simulink model "HC_core_control"  (R2023b)
settings: Solver=FixedStepAuto  StartTime=0.0  StopTime=inf  FixedStep=0.0002  RelTol=1e-4  AbsTol=1e-6
undefined symbols (not defined in the file): shuntMaxRequestedCurrentrms
settings Model: DataDictionary=fmuGenerationDictionay.sldd  ModifiedByFormat=Third Equation Ltd  Creator=Third Equation Ltd  LastModifiedBy=Third Equation Ltd
settings ConfigSet: Description=|
  | Fast task configuration for protected model and FMU generation
  | Sample frequency = 5000 Hz
settings SolverCC: AutoScaleAbsTol=off  AlgebraicLoopSolver=TrustRegion  MaxZcPerStep=1
settings DataIOCC: ExternalInput=[]  InitialState=[]  SaveFormat=Array  SaveOutput=off  SaveTime=off  ReturnWorkspaceOutputs=off
settings OptimizationCC: BlockReduction=off  BooleanDataType=off  ReuseModelBlockBuffer=off  ExpressionDepthLimit=2147483647  InitFltsAndDblsToZero=on
settings DebuggingCC: SaveWithParameterizedLinksMsg=none  SignalResolutionControl=TryResolveAllWithWarning  MultiTaskDSMMsg=warning  MultiTaskCondExecSysMsg=none  IntegerOverflowMsg=none  FcnCallInpInsideContextMsg=warning  UnconnectedInputMsg=warning  UnconnectedOutputMsg=warning  UnconnectedLineMsg=warning  StateNameClashWarn=warning  SFUnexpectedBacktrackingDiag=warning  SFNoUnconditionalDefaultTransitionDiag=warning  SFExecutionAtInitializationDiag=none  IntegerSaturationMsg=none  UnderSpecifiedDimensionMsg=warning  ArithmeticOperatorsInVariantConditions=warning
settings HardwareCC: ProdBitPerPointer=32  ProdBitPerSizeT=32  ProdBitPerPtrDiffT=32  ProdLargestAtomicFloat=None  ProdWordSize=32  ProdHWDeviceType=Custom Processor->Custom Processor
settings ModelReferenceCC: EnableRefExpFcnMdlSchedulingChecks=on  PropagateSignalLabelsOutOfModel=off
settings SFSimCC: SimUseLocalCustomCode=off  CustomCodeUndefinedFunction=UseInterfaceOnly
settings RTWCC: Description=FMU2CS  SystemTargetFile=fmu2cs.tlc  TemplateMakefile=fmu2cs_default_tmf  RTWUseLocalCustomCode=off  DLArmComputeVersion=19.05
settings CodeAppCC: StateflowObjectComments=on
settings GRTTargetCC: TargetLangStandard=C89/C90 (ANSI)  CombineOutputUpdateFcns=off  MatFileLogging=off
settings ConfigComp: CovMetricSettings=dw  CovSaveCumulativeToWorkspaceVar=on  CovSaveSingleToWorkspaceVar=on  CovExternalEMLEnable=off  CovSFcnEnable=off

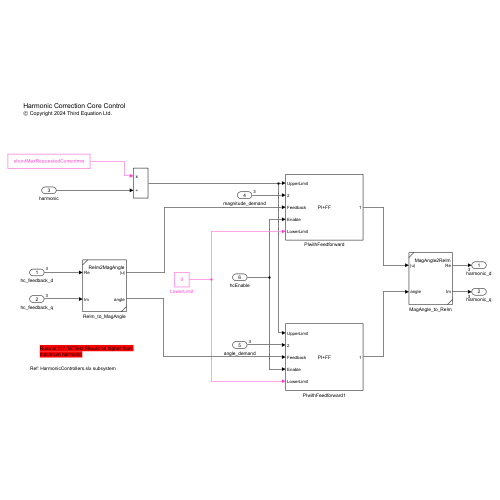
[thumbnail: Simulink's stored preview of the top-level diagram]
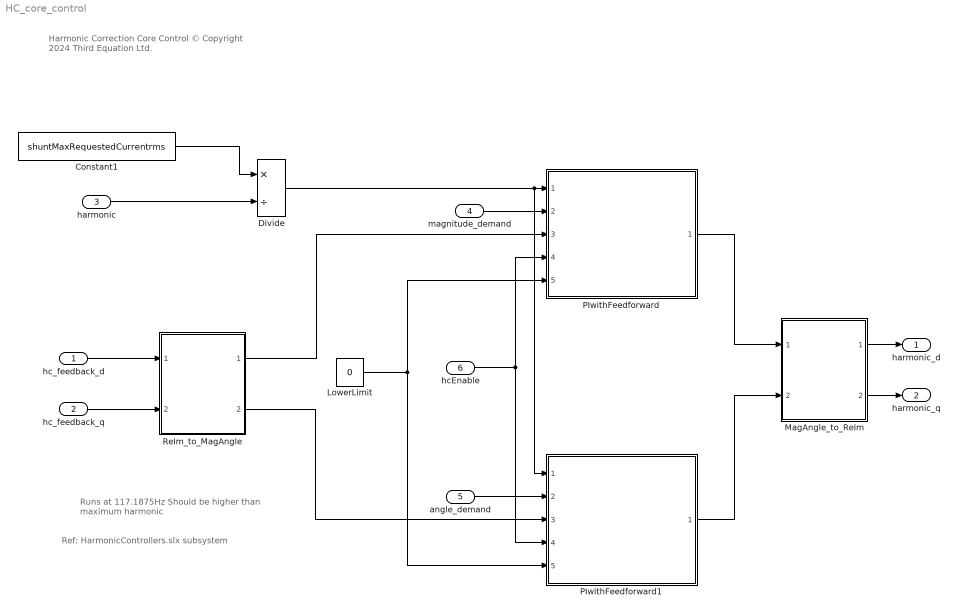
== system HC_core_control ==
  note: Ref: HarmonicControllers.slx subsystem
  note: Harmonic Correction Core Control
      | © Copyright 2024 Third Equation Ltd.
  note: Runs at 117.1875Hz Should be higher than
      | maximum harmonic
  hc_feedback_d : Inport  OutDataTypeStr=single  PortDimensions=3
  hc_feedback_q : Inport  Port=2  OutDataTypeStr=single  PortDimensions=3
  harmonic : Inport  Port=3  OutDataTypeStr=single  PortDimensions=1
  magnitude_demand : Inport  Port=4  OutDataTypeStr=single  PortDimensions=3
  angle_demand : Inport  Port=5  OutDataTypeStr=single  PortDimensions=3
  hcEnable : Inport  Port=6  OutDataTypeStr=boolean  PortDimensions=1
  Constant1 : Constant  Value=shuntMaxRequestedCurrentrms  OutDataTypeStr=single
  Divide : Product  Inputs=*/
  LowerLimit : Constant  Value=0  OutDataTypeStr=single
  MagAngle_to_ReIm : Subsystem  ReferencedSubsystem=MagAngle2ReIm
  PIwithFeedforward : Subsystem  ReferencedSubsystem=PIwithFeedforward  P=0  I=4  Gain=1
  PIwithFeedforward1 : Subsystem  ReferencedSubsystem=PIwithFeedforward  P=0  I=4  Gain=1
  ReIm_to_MagAngle : Subsystem  ReferencedSubsystem=ReIm2MagAngle
  harmonic_d : Outport  OutDataTypeStr=single  PortDimensions=3
  harmonic_q : Outport  Port=2  OutDataTypeStr=single  PortDimensions=3
  wires:
  ReIm_to_MagAngle/2 -> PIwithFeedforward1/3
  hc_feedback_q/1 -> ReIm_to_MagAngle/2
  MagAngle_to_ReIm/1 -> harmonic_d/1
  MagAngle_to_ReIm/2 -> harmonic_q/1
  hc_feedback_d/1 -> ReIm_to_MagAngle/1
  ReIm_to_MagAngle/1 -> PIwithFeedforward/3
  LowerLimit/1 -> PIwithFeedforward/5, PIwithFeedforward1/5
  PIwithFeedforward/1 -> MagAngle_to_ReIm/1
  PIwithFeedforward1/1 -> MagAngle_to_ReIm/2
  Constant1/1 -> Divide/1
  Divide/1 -> PIwithFeedforward1/1, PIwithFeedforward/1
  harmonic/1 -> Divide/2
  angle_demand/1 -> PIwithFeedforward1/2
  magnitude_demand/1 -> PIwithFeedforward/2
  hcEnable/1 -> PIwithFeedforward/4, PIwithFeedforward1/4
